simulink model "Prob_3"  (R2020b)
settings: Solver=VariableStepAuto  StartTime=0.0  StopTime=10.0  RelTol=1e-3
undefined symbols (not defined in the file or in its folder): b, m
settings Model: Creator=kshir  LastModifiedBy=kshir

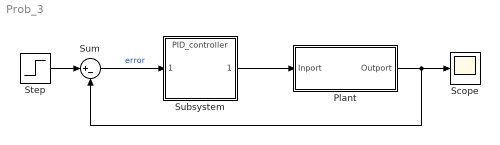
== system Prob_3 ==
  Plant : Subsystem
  Scope : Scope
  Step : Step  Time=0  After=u  SampleTime=0
  Subsystem : ModelReference  ModelNameDialog=PID_controller  SimulationMode=Normal  ModelReferenceVersion=1.3
  Sum : Sum  Inputs=|+-
  wires:
  Sum/1 -> Subsystem/1  "error"
  Step/1 -> Sum/1
  Plant/1(Outport) -> Sum/2, Scope/1
  Subsystem/1 -> Plant/1(Inport)

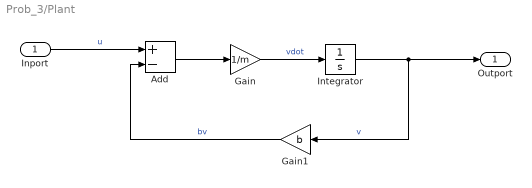
== system Prob_3/Plant ==
  Inport : Inport
  Add : Sum  Inputs=+-
  Gain : Gain  Gain=1/m
  Gain1 : Gain  Gain=b
  Integrator : Integrator
  Outport : Outport
  wires:
  Gain1/1 -> Add/2  "bv"
  Add/1 -> Gain/1
  Integrator/1 -> Outport/1, Gain1/1  "v"
  Gain/1 -> Integrator/1  "vdot"
  Inport/1 -> Add/1  "u"
